simulink model "wead"  (R2025b)
settings: Solver=FixedStepAuto  StartTime=0.0  StopTime=inf  FixedStep=0.05  RelTol=1e-3
libraries: robotlib x6
settings Model: Creator=sprinkle  LastModifiedBy=williamhenderson
settings OptimizationCC: DefaultParameterBehavior=Inlined  EnhancedBackFolding=on  PassReuseOutputArgsAs=Individual arguments  ZeroExternalMemoryAtStartup=off  ZeroInternalMemoryAtStartup=off  MaxStackSize=64  OptimizeBlockOrder=speed  DifferentSizesBufferReuse=on  OptimizationCustomize=off  EfficientTunableParamExpr=on
settings DebuggingCC: ParameterTunabilityLossMsg=error
settings HardwareCC: ProdBitPerPointer=32.0  ProdBitPerSizeT=32.0  ProdBitPerPtrDiffT=32.0  ProdLargestAtomicFloat=None  ProdIntDivRoundTo=Undefined  ProdEndianess=Unspecified  ProdWordSize=32.0  ProdHWDeviceType=Generic->Unspecified (assume 32-bit Generic)
settings SFSimCC: MATLABDynamicMemAlloc=off
settings RTWCC: SystemTargetFile=ert.tlc  HardwareBoard=Robot Operating System (ROS)  TLCOptions="-aInlineSetEventsForThisBaseRateFcn=TLC_FALSE -aSuppressMultiTaskScheduler=TLC_FALSE  -aRateBasedStepFcn=0"  GenCodeOnly=on  TemplateMakefile=ert_default_tmf  Toolchain=Catkin  TargetLang=C++  Description=Embedded Coder
settings CodeAppCC: ForceParamTrailComments=on  IgnoreCustomStorageClasses=off  OperatorAnnotations=on  SimulinkDataObjDesc=on  SFDataObjDesc=on  InsertBlockDesc=on

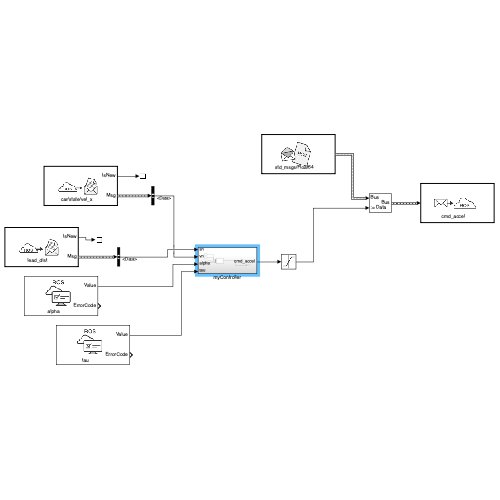
[thumbnail: Simulink's stored preview of the top-level diagram]
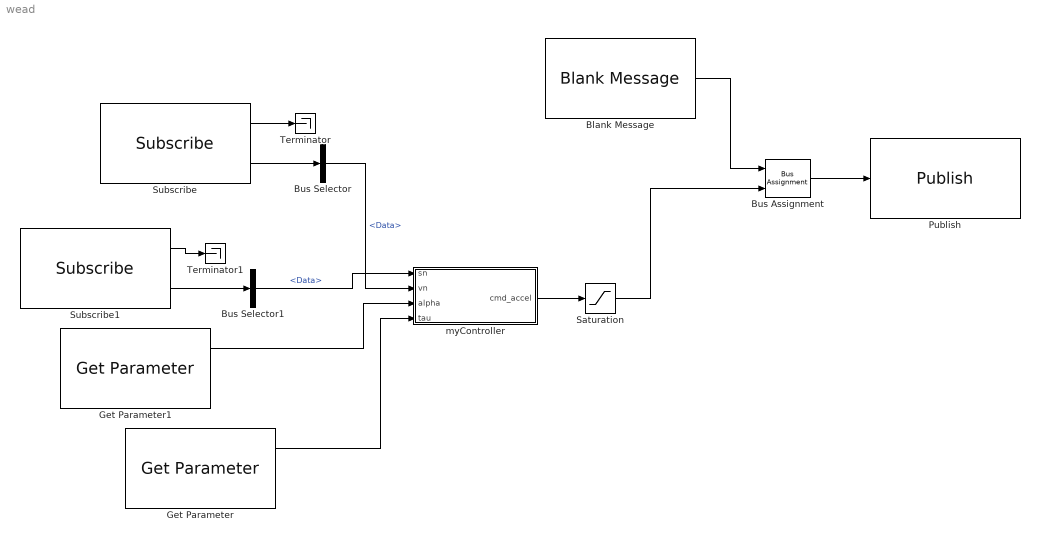
== system wead ==
  Blank Message : robotlib/Blank Message  messageClass=Message  entityType=std_msgs/Float64  messageType=std_msgs/Float64  SampleTime=inf  legacyBusStruct=off
  Bus Assignment : BusAssignment  AssignedSignals=Data
  Bus Selector : BusSelector  OutputSignals=Data
  Bus Selector1 : BusSelector  OutputSignals=Data
  Get Parameter : robotlib/Get Parameter  ParameterSource=Specify your own  ParameterName=tau  ParameterType=double  ParameterMaxArrayLength=16  ParameterInitialValue=2.0  SampleTime=-1  ShowErrorCodeOutput=on  ModelName=wead  BlockId=ParamGet_wead_18
  Get Parameter1 : robotlib/Get Parameter  ParameterSource=Specify your own  ParameterName=alpha  ParameterType=double  ParameterMaxArrayLength=16  ParameterInitialValue=1.1  SampleTime=-1  ShowErrorCodeOutput=on  ModelName=wead  BlockId=ParamGet_wead_19
  Publish : robotlib/Publish  topicSource=Specify your own  topic=cmd_accel  messageType=std_msgs/Float64  legacyBusStruct=off  messageQueueLength=1
  Saturation : Saturate  UpperLimit=1.5  LowerLimit=-3.0
  Subscribe : robotlib/Subscribe  topicSource=Specify your own  topic=car/state/vel_x  messageType=std_msgs/Float64  SampleTime=-1  legacyBusStruct=off  messageQueueLength=1
  Subscribe1 : robotlib/Subscribe  topicSource=Specify your own  topic=lead_dist  messageType=std_msgs/Float64  SampleTime=-1  legacyBusStruct=off  messageQueueLength=1
  Terminator : Terminator
  Terminator1 : Terminator
  myController : Subsystem
  wires:
  Subscribe/2 -> Bus Selector/1
  Subscribe/1 -> Terminator/1
  Subscribe1/2 -> Bus Selector1/1
  Subscribe1/1 -> Terminator1/1
  Blank Message/1 -> Bus Assignment/1
  Bus Assignment/1 -> Publish/1
  Bus Selector1/1 -> myController/1(sn)  "<Data>"
  Bus Selector/1 -> myController/2(vn)  "<Data>"
  myController/1(cmd_accel) -> Saturation/1
  Get Parameter/1 -> myController/4(tau)
  Get Parameter1/1 -> myController/3(alpha)
  Saturation/1 -> Bus Assignment/2

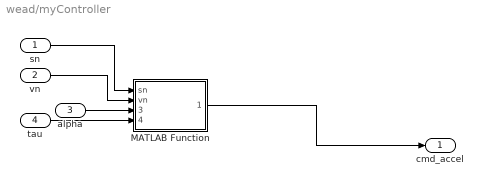
== system wead/myController ==
  sn : Inport
  vn : Inport  Port=2
  alpha : Inport  Port=3
  tau : Inport  Port=4
  MATLAB Function : MATLAB Function  TreatAsAtomicUnit=on
  cmd_accel : Outport
  wires:
  MATLAB Function/1(cmd_accel) -> cmd_accel/1
  tau/1 -> MATLAB Function/4(unused1)
  alpha/1 -> MATLAB Function/3(unused)
  sn/1 -> MATLAB Function/1(sn)
  vn/1 -> MATLAB Function/2(vn)

== matlab function wead/myController/MATLAB Function ==
  data: sn input; cmd_accel output; vn input; unused input; unused1 input
function cmd_accel = fcn(sn, vn, ~, ~)
    
    % --- Controller Tuning Parameters ---
    STOPPED_SPEED_TH = 1.0;    % [m/s] Speed threshold to be considered "stopped"
    STOPPED_MIN_GAP = 5.0;     % [m] Desired gap when stopped. Don't move if closer.
    STOPPED_ACCEL = 1.0;       % [m/s^2] Gentle acceleration from a stop
    
    MAX_ACCEL = 2.5;           % [m/s^2]
    MAX_BRAKE = -2.5;          % [m/s^2]
    
    CRUISE_SPEED_LIMIT = 36.0; % [m/s] Your speed limit
    
    % --- State 1: Stopped or Very Low Speed Logic ---
    if (vn <= STOPPED_SPEED_TH)
        % We are stopped, so we use SPACE GAP logic
        if (sn > STOPPED_MIN_GAP)
            cmd_accel = STOPPED_ACCEL; % OK to start moving
        else
            cmd_accel = 0; % Stay stopped, car in front is too close
        end
        
    else
        % --- State 2: Standard Time Gap Logic (for when vn > 1.0) ---
        time_gap = sn / vn;
    
        if (time_gap <= 3)
            % Apply full braking if gap is 3s or less
            cmd_accel = MAX_BRAKE;
        elseif (time_gap < 4)
            % Linear ramp from (3, MAX_BRAKE) to (4, 0)
            % This starts the braking process much earlier
            cmd_accel = (2.5 * time_gap) - 10;
        elseif (time_gap <= 5)
            % New "dead band" is from 4s to 5s
            cmd_accel = 0;
        elseif (time_gap < 6)
            % Linear ramp from (5, 0) to (6, MAX_ACCEL)
            cmd_accel = (2.5 * time_gap) - 12.5;
        elseif (time_gap >= 6)
            % Check cruise speed limit
            if (vn <= CRUISE_SPEED_LIMIT)
                cmd_accel = MAX_ACCEL;
            else
                cmd_accel = 0; % At cruise speed, stop accelerating
            end
        else
            % This 'else' catches all other cases (like NaN)
            % and ensures cmd_accel is always defined.
            cmd_accel = 0; % Default to a safe coasting command
        end
    end
    
end
